simulink model "P2PHVDCMMC"  (R2024a)
settings: Solver=FixedStepDiscrete  StartTime=0.0  StopTime=10  RelTol=1e-3
PreLoadFcn:
  | % HVDCMMCInterconnectionParam
StartFcn:
  | tic
StopFcn:
  | toc
values from neighbouring files (symbols this model uses):
  C_PM = 1.758e-3    (= 0.001758)    [P2PHVDCMMCcode.m]    (also in SFu.mat)
  Cg = 50e-9    (= 5e-08)    [P2PHVDCMMCcode.m]    (also in SFu.mat)
  Fc = Fnom*3.37    (= 168.5)    [P2PHVDCMMCcode.m]    (also in SFu.mat)
  Fnom = 50    [P2PHVDCMMCcode.m]    (also in SFu.mat)
  HRM = 1    [SFu.mat]
  Ki_Ireg = 6    [P2PHVDCMMCcode.m]    (also in SFu.mat)
  Ki_Preg = 1.0    (= 1)    [P2PHVDCMMCcode.m]    (also in SFu.mat)
  Ki_Qreg = 1.0    (= 1)    [P2PHVDCMMCcode.m]    (also in SFu.mat)
  Ki_VDCreg = 100    [P2PHVDCMMCcode.m]    (also in SFu.mat)
  Kp_Ireg = 0.6    [P2PHVDCMMCcode.m]    (also in SFu.mat)
  Kp_Preg = 0.5/3    (= 0.166666666667)    [P2PHVDCMMCcode.m]    (also in SFu.mat)
  Kp_Qreg = 0.5/3    (= 0.166666666667)    [P2PHVDCMMCcode.m]    (also in SFu.mat)
  Kp_VDCreg = 4    [P2PHVDCMMCcode.m]    (also in SFu.mat)
  L_cable = 15e-3    (= 0.015)    [P2PHVDCMMCcode.m]    (also in SFu.mat)
  Larm = Larm_pu*(Zb_ac/(2*pi*Fnom))    [P2PHVDCMMCcode.m]    (also in SFu.mat = 0.0529455974536)
  Larm_pu = 0.15    [P2PHVDCMMCcode.m]    (also in SFu.mat)
  Lff = Larm_pu/2    (= 0.075)    [P2PHVDCMMCcode.m]    (also in SFu.mat)
  Limits_Ireg = [ 2.0  -2.0]    [P2PHVDCMMCcode.m]    (also in SFu.mat = [2 -2])
  Limits_Preg = [ 1.2, 0.8 ]    [P2PHVDCMMCcode.m]    (also in SFu.mat = [1.2 0.8])
  Limits_Qreg = [ 0.25, -0.25 ]    [P2PHVDCMMCcode.m]    (also in SFu.mat = [0.25 -0.25])
  Limits_VDCreg = [ 2.0  -2.0]    [P2PHVDCMMCcode.m]    (also in SFu.mat = [2 -2])
  Lxfo = 0.12    [P2PHVDCMMCcode.m]    (also in SFu.mat)
  N = 1    [P2PHVDCMMCcode.m]    (also in SFu.mat)
  Nb_PM = 36    [P2PHVDCMMCcode.m]    (also in SFu.mat)
  Pnom = 1000e6    (= 1000000000)    [P2PHVDCMMCcode.m]    (also in SFu.mat)
  R_cable = 0.5    [P2PHVDCMMCcode.m]    (also in SFu.mat)
  R_startup = 400    [P2PHVDCMMCcode.m]    (also in SFu.mat)
  Rarm = Rarm_pu*Zb_ac    [P2PHVDCMMCcode.m]    (also in SFu.mat = 0.1663335)
  Rff = Rarm_pu/2    (= 0.00075)    [P2PHVDCMMCcode.m]    (also in SFu.mat)
  Rg = 100    [P2PHVDCMMCcode.m]    (also in SFu.mat)
  Rxfo = 0.003    [P2PHVDCMMCcode.m]    (also in SFu.mat)
  S =     [SFu.mat]
  Slope_Qref = 0.5    [P2PHVDCMMCcode.m]    (also in SFu.mat)
  Slope_Vdc_ref = Vnom_dc/5    (= 128000)    [P2PHVDCMMCcode.m]    (also in SFu.mat)
  Tfault = 9999    [SFu.mat]
  Ts = Ts_Control    (= 4e-05)    [P2PHVDCMMCcode.m]    (also in SFu.mat)
  Ts_Control = 40e-6    (= 4e-05)    [P2PHVDCMMCcode.m]    (also in SFu.mat)
  Ts_dqn = 2e-5    (= 2e-05)    [P2PHVDCMMCcode.m]    (also in SFu.mat)
  Ts_Power = 20e-6    (= 2e-05)    [P2PHVDCMMCcode.m]    (also in SFu.mat)
  Vnom_dc = 640e3    (= 640000)    [P2PHVDCMMCcode.m]    (also in SFu.mat)
  Vnom_prim = 400e3    (= 400000)    [P2PHVDCMMCcode.m]    (also in SFu.mat)
  Vnom_sec = 333e3    (= 333000)    [P2PHVDCMMCcode.m]    (also in SFu.mat)
  Ws = 314.159265359    [SFu.mat]
undefined symbols (not defined in the file or in its folder): DiscIntNeverNeededParam, Discrete, DQN_Lib, gcbh, Int_DQNc_Mat, Mult_DQNc_Mat, Pcc, sps, sps_rtmsupport, spsMeanValueVariableFrequencyModel, spsPLL3phModel, SY3
libraries: simulink x38, spsControlledVoltageSourceLib x30, spsVoltageMeasurementLib x21, spsIdealSwitchLib x21, powerlib_extras x12, spsSecondOrderFilterLib x12, spsCurrentMeasurementLib x12, spsdq0toabcLib x9, spsMeanLib x8, spsMeanVariableFrequencyLib x8, spsabctodq0Lib x8, spsThreePhaseSeriesRLCBranchLib x7
(part 8 of 13)

== system P2PHVDCMMC/Control _DQn_inv/PLL, Measurements and Transformation1/PLL (3ph)2/Model/Variable Frequency Mean value/Model ==
  Freq : Inport  PortDimensions=1
  vq : Inport  Port=2
  Constant : Constant  Value=1/sps.Finit
  Correction subsystem : Subsystem
  Digital Clock : DigitalClock  SampleTime=Ts
  Discrete Variable Time Delay : spsDiscreteVariableTimeDelayLib/Discrete Variable Time Delay  MaxDelay=1/sps.Fmin+Ts  InitialValue=0  Ts=Ts  DFT=on
  Gain : Gain  Gain=Ts  SaturateOnIntegerOverflow=on  OutDataTypeStr=Inherit: Same as input  ParamDataTypeStr=Inherit: Same as input
  Integ4 : DiscreteIntegrator  IntegratorMethod=Integration: Trapezoidal  SampleTime=Ts  ICPrevOutput=DiscIntNeverNeededParam  ICPrevScaledInput=DiscIntNeverNeededParam
  Number of samples per cycle : Fcn  Expr=1/u[1]/Ts
  Product : Product  InputSameDT=on  SaturateOnIntegerOverflow=on  OutDataTypeStr=Inherit: Same as first input
  Relational Operator : RelationalOperator  OutDataTypeStr=boolean  SampleTime=Ts  InputSameDT=off
  Rounding Function : Rounding  Operator=ceil
  Sum5 : Sum  InputSameDT=on  SaturateOnIntegerOverflow=on  OutDataTypeStr=Inherit: Same as first input
  Sum7 : Sum  Inputs=-+  InputSameDT=on  SaturateOnIntegerOverflow=on  OutDataTypeStr=Inherit: Same as first input
  Switch : Switch  Threshold=0.5  SaturateOnIntegerOverflow=off
  To avoid division by zero : Saturate  UpperLimit=1e6  LowerLimit=eps
  Unit Delay1 : UnitDelay  InitialCondition=sps.Vinit  SampleTime=Ts  HasFrameUpgradeWarning=on
  Mean : Outport
  wires:
  Correction subsystem/1(Out) -> Sum5/2
  To avoid division by zero/1 -> Number of samples per cycle/1  "Freq"
  Switch/1 -> Mean/1, Unit Delay1/1
  Sum5/1 -> Switch/1
  Number of samples per cycle/1 -> Correction subsystem/1(N), Rounding Function/1
  Rounding Function/1 -> Correction subsystem/2(F), Gain/1
  Gain/1 -> Discrete Variable Time Delay/2  "Delay"
  Freq/1 -> To avoid division by zero/1, Product/2
  Integ4/1 -> Sum7/2, Discrete Variable Time Delay/1
  Sum7/1 -> Product/1
  Discrete Variable Time Delay/1 -> Sum7/1
  Product/1 -> Sum5/1  "Mean value"
  vq/1 -> Correction subsystem/3(In), Integ4/1
  Digital Clock/1 -> Relational Operator/1
  Unit Delay1/1 -> Switch/3
  Relational Operator/1 -> Switch/2
  Constant/1 -> Relational Operator/2

== system P2PHVDCMMC/Control _DQn_rec/PLL, Measurements and Transformation1/PLL (3ph)/Model/Automatic Gain Control/Positive-Sequence (PLL-Driven) ==
  Freq : Inport  SampleTime=Ts
  dq : Inport  Port=2  SampleTime=Ts
  Complex to Magnitude-Angle : ComplexToMagnitudeAngle
  Mean (Variable Frequency)1 : spsMeanVariableFrequencyLib/Mean (Variable Frequency)  Finit=sps.Finit  Fmin=sps.Fmin  Vinit=sps.Real_Init  Ts=Ts
      settings: LibrarySourceBlock=|
      | sps_lib/Sensors and Measurements/Mean
      | (Variable Frequency)
  Mean (Variable Frequency)2 : spsMeanVariableFrequencyLib/Mean (Variable Frequency)  Finit=sps.Finit  Fmin=sps.Fmin  Vinit=sps.Imag_Init  Ts=Ts
      settings: LibrarySourceBlock=|
      | sps_lib/Sensors and Measurements/Mean
      | (Variable Frequency)
  Rad->Deg. : Gain  Gain=180/pi  SaturateOnIntegerOverflow=on  OutDataTypeStr=Inherit: Same as input  ParamDataTypeStr=Inherit: Same as input
  Real-Imag to Complex : RealImagToComplex
  Selector : Selector  InputPortWidth=2  IndexOptions=Index vector (dialog)  Indices=[1]  OutputSizes=1
  Selector1 : Selector  InputPortWidth=2  IndexOptions=Index vector (dialog)  Indices=[2]  OutputSizes=1
  Mag : Outport  SampleTime=Ts  VectorParamsAs1DForOutWhenUnconnected=off
  Phase : Outport  Port=2  SampleTime=Ts  VectorParamsAs1DForOutWhenUnconnected=off
  wires:
  Rad->Deg./1 -> Phase/1
  Mean (Variable Frequency)1/1 -> Real-Imag to Complex/1
  Freq/1 -> Mean (Variable Frequency)1/1, Mean (Variable Frequency)2/1
  Real-Imag to Complex/1 -> Complex to Magnitude-Angle/1
  Mean (Variable Frequency)2/1 -> Real-Imag to Complex/2
  Complex to Magnitude-Angle/1 -> Mag/1
  Complex to Magnitude-Angle/2 -> Rad->Deg./1
  dq/1 -> Selector/1, Selector1/1  "q"
  Selector/1 -> Mean (Variable Frequency)1/2  "d"
  Selector1/1 -> Mean (Variable Frequency)2/2  "q"

== system P2PHVDCMMC/Control _DQn_rec/PLL, Measurements and Transformation1/PLL (3ph)/Model/Variable Frequency Mean value/Model ==
  Freq : Inport  PortDimensions=1
  vq : Inport  Port=2
  Constant : Constant  Value=1/sps.Finit
  Correction subsystem : Subsystem
  Digital Clock : DigitalClock  SampleTime=Ts
  Discrete Variable Time Delay : spsDiscreteVariableTimeDelayLib/Discrete Variable Time Delay  MaxDelay=1/sps.Fmin+Ts  InitialValue=0  Ts=Ts  DFT=on
  Gain : Gain  Gain=Ts  SaturateOnIntegerOverflow=on  OutDataTypeStr=Inherit: Same as input  ParamDataTypeStr=Inherit: Same as input
  Integ4 : DiscreteIntegrator  IntegratorMethod=Integration: Trapezoidal  SampleTime=Ts  ICPrevOutput=DiscIntNeverNeededParam  ICPrevScaledInput=DiscIntNeverNeededParam
  Number of samples per cycle : Fcn  Expr=1/u[1]/Ts
  Product : Product  InputSameDT=on  SaturateOnIntegerOverflow=on  OutDataTypeStr=Inherit: Same as first input
  Relational Operator : RelationalOperator  OutDataTypeStr=boolean  SampleTime=Ts  InputSameDT=off
  Rounding Function : Rounding  Operator=ceil
  Sum5 : Sum  InputSameDT=on  SaturateOnIntegerOverflow=on  OutDataTypeStr=Inherit: Same as first input
  Sum7 : Sum  Inputs=-+  InputSameDT=on  SaturateOnIntegerOverflow=on  OutDataTypeStr=Inherit: Same as first input
  Switch : Switch  Threshold=0.5  SaturateOnIntegerOverflow=off
  To avoid division by zero : Saturate  UpperLimit=1e6  LowerLimit=eps
  Unit Delay1 : UnitDelay  InitialCondition=sps.Vinit  SampleTime=Ts  HasFrameUpgradeWarning=on
  Mean : Outport
  wires:
  Correction subsystem/1(Out) -> Sum5/2
  To avoid division by zero/1 -> Number of samples per cycle/1  "Freq"
  Switch/1 -> Mean/1, Unit Delay1/1
  Sum5/1 -> Switch/1
  Number of samples per cycle/1 -> Correction subsystem/1(N), Rounding Function/1
  Rounding Function/1 -> Correction subsystem/2(F), Gain/1
  Gain/1 -> Discrete Variable Time Delay/2  "Delay"
  Freq/1 -> To avoid division by zero/1, Product/2
  Integ4/1 -> Sum7/2, Discrete Variable Time Delay/1
  Sum7/1 -> Product/1
  Discrete Variable Time Delay/1 -> Sum7/1
  Product/1 -> Sum5/1  "Mean value"
  vq/1 -> Correction subsystem/3(In), Integ4/1
  Digital Clock/1 -> Relational Operator/1
  Unit Delay1/1 -> Switch/3
  Relational Operator/1 -> Switch/2
  Constant/1 -> Relational Operator/2

== system P2PHVDCMMC/Control _DQn_rec/PLL, Measurements and Transformation1/PLL (3ph)2/Model/Automatic Gain Control/Positive-Sequence (PLL-Driven) ==
  Freq : Inport  SampleTime=Ts
  dq : Inport  Port=2  SampleTime=Ts
  Complex to Magnitude-Angle : ComplexToMagnitudeAngle
  Mean (Variable Frequency)1 : spsMeanVariableFrequencyLib/Mean (Variable Frequency)  Finit=sps.Finit  Fmin=sps.Fmin  Vinit=sps.Real_Init  Ts=Ts
      settings: LibrarySourceBlock=|
      | sps_lib/Sensors and Measurements/Mean
      | (Variable Frequency)
  Mean (Variable Frequency)2 : spsMeanVariableFrequencyLib/Mean (Variable Frequency)  Finit=sps.Finit  Fmin=sps.Fmin  Vinit=sps.Imag_Init  Ts=Ts
      settings: LibrarySourceBlock=|
      | sps_lib/Sensors and Measurements/Mean
      | (Variable Frequency)
  Rad->Deg. : Gain  Gain=180/pi  SaturateOnIntegerOverflow=on  OutDataTypeStr=Inherit: Same as input  ParamDataTypeStr=Inherit: Same as input
  Real-Imag to Complex : RealImagToComplex
  Selector : Selector  InputPortWidth=2  IndexOptions=Index vector (dialog)  Indices=[1]  OutputSizes=1
  Selector1 : Selector  InputPortWidth=2  IndexOptions=Index vector (dialog)  Indices=[2]  OutputSizes=1
  Mag : Outport  SampleTime=Ts  VectorParamsAs1DForOutWhenUnconnected=off
  Phase : Outport  Port=2  SampleTime=Ts  VectorParamsAs1DForOutWhenUnconnected=off
  wires:
  Rad->Deg./1 -> Phase/1
  Mean (Variable Frequency)1/1 -> Real-Imag to Complex/1
  Freq/1 -> Mean (Variable Frequency)1/1, Mean (Variable Frequency)2/1
  Real-Imag to Complex/1 -> Complex to Magnitude-Angle/1
  Mean (Variable Frequency)2/1 -> Real-Imag to Complex/2
  Complex to Magnitude-Angle/1 -> Mag/1
  Complex to Magnitude-Angle/2 -> Rad->Deg./1
  dq/1 -> Selector/1, Selector1/1  "q"
  Selector/1 -> Mean (Variable Frequency)1/2  "d"
  Selector1/1 -> Mean (Variable Frequency)2/2  "q"

== system P2PHVDCMMC/Control _DQn_rec/PLL, Measurements and Transformation1/PLL (3ph)2/Model/Variable Frequency Mean value/Model ==
  Freq : Inport  PortDimensions=1
  vq : Inport  Port=2
  Constant : Constant  Value=1/sps.Finit
  Correction subsystem : Subsystem
  Digital Clock : DigitalClock  SampleTime=Ts
  Discrete Variable Time Delay : spsDiscreteVariableTimeDelayLib/Discrete Variable Time Delay  MaxDelay=1/sps.Fmin+Ts  InitialValue=0  Ts=Ts  DFT=on
  Gain : Gain  Gain=Ts  SaturateOnIntegerOverflow=on  OutDataTypeStr=Inherit: Same as input  ParamDataTypeStr=Inherit: Same as input
  Integ4 : DiscreteIntegrator  IntegratorMethod=Integration: Trapezoidal  SampleTime=Ts  ICPrevOutput=DiscIntNeverNeededParam  ICPrevScaledInput=DiscIntNeverNeededParam
  Number of samples per cycle : Fcn  Expr=1/u[1]/Ts
  Product : Product  InputSameDT=on  SaturateOnIntegerOverflow=on  OutDataTypeStr=Inherit: Same as first input
  Relational Operator : RelationalOperator  OutDataTypeStr=boolean  SampleTime=Ts  InputSameDT=off
  Rounding Function : Rounding  Operator=ceil
  Sum5 : Sum  InputSameDT=on  SaturateOnIntegerOverflow=on  OutDataTypeStr=Inherit: Same as first input
  Sum7 : Sum  Inputs=-+  InputSameDT=on  SaturateOnIntegerOverflow=on  OutDataTypeStr=Inherit: Same as first input
  Switch : Switch  Threshold=0.5  SaturateOnIntegerOverflow=off
  To avoid division by zero : Saturate  UpperLimit=1e6  LowerLimit=eps
  Unit Delay1 : UnitDelay  InitialCondition=sps.Vinit  SampleTime=Ts  HasFrameUpgradeWarning=on
  Mean : Outport
  wires:
  Correction subsystem/1(Out) -> Sum5/2
  To avoid division by zero/1 -> Number of samples per cycle/1  "Freq"
  Switch/1 -> Mean/1, Unit Delay1/1
  Sum5/1 -> Switch/1
  Number of samples per cycle/1 -> Correction subsystem/1(N), Rounding Function/1
  Rounding Function/1 -> Correction subsystem/2(F), Gain/1
  Gain/1 -> Discrete Variable Time Delay/2  "Delay"
  Freq/1 -> To avoid division by zero/1, Product/2
  Integ4/1 -> Sum7/2, Discrete Variable Time Delay/1
  Sum7/1 -> Product/1
  Discrete Variable Time Delay/1 -> Sum7/1
  Product/1 -> Sum5/1  "Mean value"
  vq/1 -> Correction subsystem/3(In), Integ4/1
  Digital Clock/1 -> Relational Operator/1
  Unit Delay1/1 -> Switch/3
  Relational Operator/1 -> Switch/2
  Constant/1 -> Relational Operator/2

== system P2PHVDCMMC/Control _DQn_inv/PLL, Measurements and Transformation1/PLL (3ph)/Model/Variable Frequency Mean value/Model/Correction subsystem ==
  N : Inport
  F : Inport  Port=2
  In : Inport  Port=3
  Gain1 : Gain  Gain=0.5  SaturateOnIntegerOverflow=on  OutDataTypeStr=Inherit: Same as input  ParamDataTypeStr=Inherit: Same as input
  Product2 : Product  Inputs=*/  InputSameDT=on  SaturateOnIntegerOverflow=on  OutDataTypeStr=Inherit: Same as first input
  Product4 : Product  Inputs=**  InputSameDT=on  SaturateOnIntegerOverflow=on  OutDataTypeStr=Inherit: Same as first input
  Product5 : Product  Inputs=**  InputSameDT=on  SaturateOnIntegerOverflow=on  OutDataTypeStr=Inherit: Same as first input
  Sum1 : Sum  Inputs=+-  InputSameDT=on  SaturateOnIntegerOverflow=on  OutDataTypeStr=Inherit: Same as first input
  Sum4 : Sum  InputSameDT=on  SaturateOnIntegerOverflow=on  OutDataTypeStr=Inherit: Same as first input
  Sum5 : Sum  Inputs=+-  InputSameDT=on  SaturateOnIntegerOverflow=on  OutDataTypeStr=Inherit: Same as first input
  Unit Delay : UnitDelay  SampleTime=Ts  HasFrameUpgradeWarning=on
  Out : Outport
  wires:
  Product4/1 -> Out/1
  Sum4/1 -> Product4/2
  Gain1/1 -> Sum4/1
  Product5/1 -> Gain1/1
  Sum1/1 -> Product5/2
  In/1 -> Sum4/2, Unit Delay/1, Sum1/1
  Product2/1 -> Product4/1
  Sum5/1 -> Product5/1, Product2/1
  F/1 -> Sum5/2
  N/1 -> Product2/2, Sum5/1
  Unit Delay/1 -> Sum1/2

== system P2PHVDCMMC/Control _DQn_inv/PLL, Measurements and Transformation1/PLL (3ph)2/Model/Variable Frequency Mean value/Model/Correction subsystem ==
  N : Inport
  F : Inport  Port=2
  In : Inport  Port=3
  Gain1 : Gain  Gain=0.5  SaturateOnIntegerOverflow=on  OutDataTypeStr=Inherit: Same as input  ParamDataTypeStr=Inherit: Same as input
  Product2 : Product  Inputs=*/  InputSameDT=on  SaturateOnIntegerOverflow=on  OutDataTypeStr=Inherit: Same as first input
  Product4 : Product  Inputs=**  InputSameDT=on  SaturateOnIntegerOverflow=on  OutDataTypeStr=Inherit: Same as first input
  Product5 : Product  Inputs=**  InputSameDT=on  SaturateOnIntegerOverflow=on  OutDataTypeStr=Inherit: Same as first input
  Sum1 : Sum  Inputs=+-  InputSameDT=on  SaturateOnIntegerOverflow=on  OutDataTypeStr=Inherit: Same as first input
  Sum4 : Sum  InputSameDT=on  SaturateOnIntegerOverflow=on  OutDataTypeStr=Inherit: Same as first input
  Sum5 : Sum  Inputs=+-  InputSameDT=on  SaturateOnIntegerOverflow=on  OutDataTypeStr=Inherit: Same as first input
  Unit Delay : UnitDelay  SampleTime=Ts  HasFrameUpgradeWarning=on
  Out : Outport
  wires:
  Product4/1 -> Out/1
  Sum4/1 -> Product4/2
  Gain1/1 -> Sum4/1
  Product5/1 -> Gain1/1
  Sum1/1 -> Product5/2
  In/1 -> Sum4/2, Unit Delay/1, Sum1/1
  Product2/1 -> Product4/1
  Sum5/1 -> Product5/1, Product2/1
  F/1 -> Sum5/2
  N/1 -> Product2/2, Sum5/1
  Unit Delay/1 -> Sum1/2

== system P2PHVDCMMC/Control _DQn_rec/PLL, Measurements and Transformation1/PLL (3ph)/Model/Variable Frequency Mean value/Model/Correction subsystem ==
  N : Inport
  F : Inport  Port=2
  In : Inport  Port=3
  Gain1 : Gain  Gain=0.5  SaturateOnIntegerOverflow=on  OutDataTypeStr=Inherit: Same as input  ParamDataTypeStr=Inherit: Same as input
  Product2 : Product  Inputs=*/  InputSameDT=on  SaturateOnIntegerOverflow=on  OutDataTypeStr=Inherit: Same as first input
  Product4 : Product  Inputs=**  InputSameDT=on  SaturateOnIntegerOverflow=on  OutDataTypeStr=Inherit: Same as first input
  Product5 : Product  Inputs=**  InputSameDT=on  SaturateOnIntegerOverflow=on  OutDataTypeStr=Inherit: Same as first input
  Sum1 : Sum  Inputs=+-  InputSameDT=on  SaturateOnIntegerOverflow=on  OutDataTypeStr=Inherit: Same as first input
  Sum4 : Sum  InputSameDT=on  SaturateOnIntegerOverflow=on  OutDataTypeStr=Inherit: Same as first input
  Sum5 : Sum  Inputs=+-  InputSameDT=on  SaturateOnIntegerOverflow=on  OutDataTypeStr=Inherit: Same as first input
  Unit Delay : UnitDelay  SampleTime=Ts  HasFrameUpgradeWarning=on
  Out : Outport
  wires:
  Product4/1 -> Out/1
  Sum4/1 -> Product4/2
  Gain1/1 -> Sum4/1
  Product5/1 -> Gain1/1
  Sum1/1 -> Product5/2
  In/1 -> Sum4/2, Unit Delay/1, Sum1/1
  Product2/1 -> Product4/1
  Sum5/1 -> Product5/1, Product2/1
  F/1 -> Sum5/2
  N/1 -> Product2/2, Sum5/1
  Unit Delay/1 -> Sum1/2

== system P2PHVDCMMC/Control _DQn_rec/PLL, Measurements and Transformation1/PLL (3ph)2/Model/Variable Frequency Mean value/Model/Correction subsystem ==
  N : Inport
  F : Inport  Port=2
  In : Inport  Port=3
  Gain1 : Gain  Gain=0.5  SaturateOnIntegerOverflow=on  OutDataTypeStr=Inherit: Same as input  ParamDataTypeStr=Inherit: Same as input
  Product2 : Product  Inputs=*/  InputSameDT=on  SaturateOnIntegerOverflow=on  OutDataTypeStr=Inherit: Same as first input
  Product4 : Product  Inputs=**  InputSameDT=on  SaturateOnIntegerOverflow=on  OutDataTypeStr=Inherit: Same as first input
  Product5 : Product  Inputs=**  InputSameDT=on  SaturateOnIntegerOverflow=on  OutDataTypeStr=Inherit: Same as first input
  Sum1 : Sum  Inputs=+-  InputSameDT=on  SaturateOnIntegerOverflow=on  OutDataTypeStr=Inherit: Same as first input
  Sum4 : Sum  InputSameDT=on  SaturateOnIntegerOverflow=on  OutDataTypeStr=Inherit: Same as first input
  Sum5 : Sum  Inputs=+-  InputSameDT=on  SaturateOnIntegerOverflow=on  OutDataTypeStr=Inherit: Same as first input
  Unit Delay : UnitDelay  SampleTime=Ts  HasFrameUpgradeWarning=on
  Out : Outport
  wires:
  Product4/1 -> Out/1
  Sum4/1 -> Product4/2
  Gain1/1 -> Sum4/1
  Product5/1 -> Gain1/1
  Sum1/1 -> Product5/2
  In/1 -> Sum4/2, Unit Delay/1, Sum1/1
  Product2/1 -> Product4/1
  Sum5/1 -> Product5/1, Product2/1
  F/1 -> Sum5/2
  N/1 -> Product2/2, Sum5/1
  Unit Delay/1 -> Sum1/2

== matlab function P2PHVDCMMC/Subsystem4/ACrec/Mult_DQNc_Mat2 ==
  data: Xdcpnz_c input; Ydcpnz_c input; N parameter; HrmDbl parameter; Zdcpnz_c output
function Zdcpnz_c    = fMultDQNc(Xdcpnz_c, Ydcpnz_c, N, HrmDbl)
    Zdcpnz_c = complex(zeros(3,2*N+1));

    persistent T132;
    persistent T213;
    persistent T231;
    persistent T321;
    persistent T312;
    persistent Sas;
    persistent Ssa;

    if(isempty(T132)) 
        T132 = [1 0 0; 0 0 1; 0 1 0];
        T213 = [0 1 0; 1 0 0; 0 0 1];
        T231 = [0 1 0; 0 0 1; 1 0 0];
        T321 = [0 0 1; 0 1 0; 1 0 0];
        T312 = [0 0 1; 1 0 0; 0 1 0];

        a = -0.5+0.866i;
        a2 = -0.5-0.866i;
        Sas = [1,a,a2;1,a2,a;1,1,1]/3;
        Ssa = eye(3)/(Sas);
    end

%%%%%%%%%%%%%%%%%%%%%%%%%%%%%%

    Zdcpnz_c(:,1) = Sas*(Ssa*Xdcpnz_c(:,1).*Ssa*Ydcpnz_c(:,1));

    sX = size(Xdcpnz_c,2);
    Xdcpnz_c = [Xdcpnz_c zeros(3,N+1-sX)];

    sY = size(Ydcpnz_c,2);
    Ydcpnz_c = [Ydcpnz_c zeros(3,N+1-sY)];

       
    for h = 1 : 2*N
        if(h<=N)

            Zdcpnz_c(3,1) = Zdcpnz_c(3,1) + 0.5*real(Xdcpnz_c(:,h+1)'*Ydcpnz_c(:,h+1));


            Zdcpnz_c(3,2*h+1) = Zdcpnz_c(3,2*h+1) + 0.5*Xdcpnz_c(1,h+1)*Ydcpnz_c(2,h+1)*exp(-1i*pi/2);

            Zdcpnz_c(1:2,1) = Zdcpnz_c(1:2,1) + 0.25*abs(Xdcpnz_c(1,h+1))*abs(Ydcpnz_c(2,h+1))*[1;1].*exp(1i*((-angle(Xdcpnz_c(1,h+1))+angle(Ydcpnz_c(2,h+1)))*[1;-1]));
            Zdcpnz_c(1:2,1) = Zdcpnz_c(1:2,1) + 0.25*abs(Xdcpnz_c(1,h+1))*abs(Ydcpnz_c(3,h+1))*[1;1].*exp(1i*((-angle(Xdcpnz_c(1,h+1))+angle(Ydcpnz_c(3,h+1)))*[-1;1]));


            Zdcpnz_c(3,2*h+1) = Zdcpnz_c(3,2*h+1) + 0.5*Xdcpnz_c(2,h+1)*Ydcpnz_c(1,h+1)*exp(-1i*pi/2);


            Zdcpnz_c(1:2,1) = Zdcpnz_c(1:2,1) + 0.25*abs(Xdcpnz_c(2,h+1))*abs(Ydcpnz_c(1,h+1))*[1;1].*exp(1i*((-angle(Xdcpnz_c(2,h+1))+angle(Ydcpnz_c(1,h+1)))*[-1;1]));
            Zdcpnz_c(1:2,1) = Zdcpnz_c(1:2,1) + 0.25*abs(Xdcpnz_c(2,h+1))*abs(Ydcpnz_c(3,h+1))*[1;1].*exp(1i*((-angle(Xdcpnz_c(2,h+1))+angle(Ydcpnz_c(3,h+1)))*[1;-1]));
            
            Zdcpnz_c(1:2,1) = Zdcpnz_c(1:2,1) + 0.25*abs(Xdcpnz_c(3,h+1))*abs(Ydcpnz_c(1,h+1))*[1;1].*exp(1i*((-angle(Xdcpnz_c(3,h+1))+angle(Ydcpnz_c(1,h+1)))*[1;-1]));
            Zdcpnz_c(1:2,1) = Zdcpnz_c(1:2,1) + 0.25*abs(Xdcpnz_c(3,h+1))*abs(Ydcpnz_c(2,h+1))*[1;1].*exp(1i*((-angle(Xdcpnz_c(3,h+1))+angle(Ydcpnz_c(2,h+1)))*[-1;+1]));

            %%%%%%%%%%%%%%%%% POSITIVE (Ydc*Xp) %%%%%%%%%%%%%%%%%%%
            Zdcpnz_c(:,h+1) = Zdcpnz_c(:,h+1) + T312*Ydcpnz_c(:,1)*Xdcpnz_c(1,h+1); %[0 0 1; 1 0 0; 0 1 0]
            %%%%%%%%%%%%%%%%% POSITIVE (Xdc*Yp) %%%%%%%%%%%%%%%%%%%
            Zdcpnz_c(:,h+1) = Zdcpnz_c(:,h+1) + T312*Xdcpnz_c(:,1)*Ydcpnz_c(1,h+1);
            %%%%%%%%%%%%%%%%% NEGATIVE (Ydc*Xn) %%%%%%%%%%%%%%%%%%%
            Zdcpnz_c(:,h+1) = Zdcpnz_c(:,h+1) + T231*Ydcpnz_c(:,1)*Xdcpnz_c(2,h+1);
            %%%%%%%%%%%%%%%%% NEGATIVE (Xdc*Yn) %%%%%%%%%%%%%%%%%%%
            Zdcpnz_c(:,h+1) = Zdcpnz_c(:,h+1) + T231*Xdcpnz_c(:,1)*Ydcpnz_c(2,h+1);
            %%%%%%%%%%%%%%%%%%%%%%%%%%%%%%%%%%%%%%%%%%%%%%%%%%%%%%
            Zdcpnz_c(:,h+1) = Zdcpnz_c(:,h+1) + Ydcpnz_c(:,1)*Xdcpnz_c(3,h+1);
            %%%%%%%%%%%%%%%%%%%%%%%%%%%%%%%%%%%%%%%%%%%%%%%%%%%%%%
            Zdcpnz_c(:,h+1) = Zdcpnz_c(:,h+1) + Xdcpnz_c(:,1)*Ydcpnz_c(3,h+1);
            
%%%%%%%%%%%%%%%%%%%%%% h<=N ODD %%%%%%%%%%%%%%%%%%%%%%%%%%%%%%%%%%%%%%%%%
            if(mod(h,2)==1) 
                %%%%%%%%%%%%%%%%% D3p (3ph+) %%%%%%%%%%%%%%%%%%%%%%%

                %&%%%%%%%%%%%%%%%%%%%%%%%%%% PP + NN %%%%%%%%%%%%%%%%%%%%%%%%%%%
                for i = 1 : h - 1
                   Zdcpnz_c(1,h+1) = Zdcpnz_c(1,h+1) +    0.5*( real(Xdcpnz_c(2,i+1))*imag(Ydcpnz_c(2,h-i+1)) + imag(Xdcpnz_c(2,i+1))*real(Ydcpnz_c(2,h-i+1)) );
                   Zdcpnz_c(1,h+1) = Zdcpnz_c(1,h+1) + 1i*0.5*( -real(Xdcpnz_c(2,i+1))*real(Ydcpnz_c(2,h-i+1)) + imag(Xdcpnz_c(2,i+1))*imag(Ydcpnz_c(2,h-i+1)) );

                   Zdcpnz_c(2,h+1) = Zdcpnz_c(2,h+1) +    0.5*( real(Xdcpnz_c(1,i+1))*imag(Ydcpnz_c(1,h-i+1)) + imag(Xdcpnz_c(1,i+1))*real(Ydcpnz_c(1,h-i+1)) );
                   Zdcpnz_c(2,h+1) = Zdcpnz_c(2,h+1) + 1i*0.5*( -real(Xdcpnz_c(1,i+1))*real(Ydcpnz_c(1,h-i+1)) + imag(Xdcpnz_c(1,i+1))*imag(Ydcpnz_c(1,h-i+1)) );
                end

                for i = 1 : N - h

                    Zdcpnz_c(3,h+1) = Zdcpnz_c(3,h+1) -    imag(0.5*Xdcpnz_c(1:2,i+1)'*Ydcpnz_c(1:2,i+h+1)) -    imag(0.5*Ydcpnz_c(1:2,i+1)'*Xdcpnz_c(1:2,i+h+1));
                    Zdcpnz_c(3,h+1) = Zdcpnz_c(3,h+1) + 1i*real(0.5*Xdcpnz_c(1:2,i+1)'*Ydcpnz_c(1:2,i+h+1)) + 1i*real(0.5*Ydcpnz_c(1:2,i+1)'*Xdcpnz_c(1:2,i+h+1));

                end
                %&%%%%%%%%%%%%%%%%%%%%%%%%%% PP + NN %%%%%%%%%%%%%%%%%%%%%%%%%%%

                for k = 1 : (N + mod(N+1,2) - h)/2
                    i = 2*k-1;
                    j = i+h;

                    Zdcpnz_c(1,h+1) = Zdcpnz_c(1,h+1) + (0.5*(Xdcpnz_c(:,i+1)'*T132*T213*Ydcpnz_c(:,j+1))*exp(+1i*pi/2)) ...
                                                      + (0.5*(Xdcpnz_c(:,j+1)'*T213*T132*Ydcpnz_c(:,i+1))*exp(-1i*pi/2))';

                    Zdcpnz_c(2,h+1) = Zdcpnz_c(2,h+1) + (0.5*(Xdcpnz_c(:,i+1)'*T132*T321*Ydcpnz_c(:,j+1))*exp(+1i*pi/2)) ...
                                                      + (0.5*(Xdcpnz_c(:,j+1)'*T321*T132*Ydcpnz_c(:,i+1))*exp(-1i*pi/2))';

                    Zdcpnz_c(3,h+1) = Zdcpnz_c(3,h+1) + (0.5*Xdcpnz_c(3,i+1)'*Ydcpnz_c(3,j+1)*exp(1i*pi/2)) ...
                                                      - (0.5*Xdcpnz_c(3,j+1)'*Ydcpnz_c(3,i+1)*exp(1i*pi/2))';
                end

                for k = 1 : (N + mod(N,2) - h - 1)/2
                    i = 2*k;
                    j = i+h;
                    
                    Zdcpnz_c(1,h+1) = Zdcpnz_c(1,h+1) + (0.5*(Xdcpnz_c(:,i+1)'*T132*T213*Ydcpnz_c(:,j+1))*exp(+1i*pi/2)) ...
                                                      + (0.5*(Xdcpnz_c(:,j+1)'*T213*T132*Ydcpnz_c(:,i+1))*exp(-1i*pi/2))';

                    Zdcpnz_c(2,h+1) = Zdcpnz_c(2,h+1) + (0.5*(Xdcpnz_c(:,i+1)'*T132*T321*Ydcpnz_c(:,j+1))*exp(+1i*pi/2)) ...
                                                      + (0.5*(Xdcpnz_c(:,j+1)'*T321*T132*Ydcpnz_c(:,i+1))*exp(-1i*pi/2))';

                    Zdcpnz_c(3,h+1) = Zdcpnz_c(3,h+1) + (0.5*Xdcpnz_c(3,i+1)'*Ydcpnz_c(3,j+1)*exp(1i*pi/2)) ...
                                                      - (0.5*Xdcpnz_c(3,j+1)'*Ydcpnz_c(3,i+1)*exp(1i*pi/2))';
                end

                for k = (h-1)/2:-1:1
                    i = k;
                    j = h-i;  

                    Zdcpnz_c(3,h+1) = Zdcpnz_c(3,h+1) + 0.5*(real(Xdcpnz_c(:,i+1))'*T213*imag(Ydcpnz_c(:,j+1)) + imag(Xdcpnz_c(:,i+1))'*T213*real(Ydcpnz_c(:,j+1)) ...
                                                           + real(Xdcpnz_c(:,j+1))'*T213*imag(Ydcpnz_c(:,i+1)) + imag(Xdcpnz_c(:,j+1))'*T213*real(Ydcpnz_c(:,i+1)));
                                                                                       
                    Zdcpnz_c(3,h+1) = Zdcpnz_c(3,h+1) + 1i*0.5*(-real(Xdcpnz_c(:,i+1))'*T213*real(Ydcpnz_c(:,j+1)) + imag(Xdcpnz_c(:,i+1))'*T213*imag(Ydcpnz_c(:,j+1)) ...
                                                           - real(Xdcpnz_c(:,j+1))'*T213*real(Ydcpnz_c(:,i+1)) + imag(Xdcpnz_c(:,j+1))'*T213*imag(Ydcpnz_c(:,i+1)));

                    Zdcpnz_c(1,h+1) = Zdcpnz_c(1,h+1) + 0.5*(real(Xdcpnz_c([1,3],i+1))'*[0 1; 1 0]*imag(Ydcpnz_c([1,3],j+1)) + imag(Xdcpnz_c([1,3],i+1))'*[0 1; 1 0]*real(Ydcpnz_c([1,3],j+1)) ...
                                                           + real(Xdcpnz_c([1,3],j+1))'*[0 1; 1 0]*imag(Ydcpnz_c([1,3],i+1)) + imag(Xdcpnz_c([1,3],j+1))'*[0 1; 1 0]*real(Ydcpnz_c([1,3],i+1)) );

                    Zdcpnz_c(1,h+1) = Zdcpnz_c(1,h+1) + 1i*0.5*(-real(Xdcpnz_c([1,3],i+1))'*[0 1; 1 0]*real(Ydcpnz_c([1,3],j+1)) + imag(Xdcpnz_c([1,3],i+1))'*[0 1; 1 0]*imag(Ydcpnz_c([1,3],j+1)) ...
                                                              - real(Xdcpnz_c([1,3],j+1))'*[0 1; 1 0]*real(Ydcpnz_c([1,3],i+1)) + imag(Xdcpnz_c([1,3],j+1))'*[0 1; 1 0]*imag(Ydcpnz_c([1,3],i+1)) );

                    Zdcpnz_c(2,h+1) = Zdcpnz_c(2,h+1) + 0.5*(real(Xdcpnz_c([2,3],i+1))'*[0 1; 1 0]*imag(Ydcpnz_c([2,3],j+1)) + imag(Xdcpnz_c([2,3],i+1))'*[0 1; 1 0]*real(Ydcpnz_c([2,3],j+1)) ...
                                                           + real(Xdcpnz_c([2,3],j+1))'*[0 1; 1 0]*imag(Ydcpnz_c([2,3],i+1)) + imag(Xdcpnz_c([2,3],j+1))'*[0 1; 1 0]*real(Ydcpnz_c([2,3],i+1)) );

                    Zdcpnz_c(2,h+1) = Zdcpnz_c(2,h+1) + 1i*0.5*(-real(Xdcpnz_c([2,3],i+1))'*[0 1; 1 0]*real(Ydcpnz_c([2,3],j+1)) + imag(Xdcpnz_c([2,3],i+1))'*[0 1; 1 0]*imag(Ydcpnz_c([2,3],j+1)) ...
                                                              - real(Xdcpnz_c([2,3],j+1))'*[0 1; 1 0]*real(Ydcpnz_c([2,3],i+1)) + imag(Xdcpnz_c([2,3],j+1))'*[0 1; 1 0]*imag(Ydcpnz_c([2,3],i+1)) );

                end
%%%%%%%%%%%%%%%%%%%%%% h<=N EVEN %%%%%%%%%%%%%%%%%%%%%%%%%%%%%%%%%%%%%%%%%           
            else  

                Zdcpnz_c(3,h+1) = Zdcpnz_c(3,h+1) + 0.5*imag(Xdcpnz_c(3,h/2+1)*Ydcpnz_c(3,h/2+1))           -0.5*1i*real(Xdcpnz_c(3,h/2+1)*Ydcpnz_c(3,h/2+1));
                Zdcpnz_c(1,h+1) = Zdcpnz_c(1,h+1) + 0.5*real(Xdcpnz_c(:,h/2+1))'*T321*imag(Ydcpnz_c(:,h/2+1)) + 0.5*imag(Xdcpnz_c(:,h/2+1))'*T321*real(Ydcpnz_c(:,h/2+1));
                Zdcpnz_c(1,h+1) = Zdcpnz_c(1,h+1) - 0.5*1i*real(Xdcpnz_c(:,h/2+1))'*T321*real(Ydcpnz_c(:,h/2+1)) + 0.5*1i*imag(Xdcpnz_c(:,h/2+1))'*T321*imag(Ydcpnz_c(:,h/2+1));
                Zdcpnz_c(2,h+1) = Zdcpnz_c(2,h+1) + 0.5*real(Xdcpnz_c(:,h/2+1))'*T132*imag(Ydcpnz_c(:,h/2+1)) + 0.5*imag(Xdcpnz_c(:,h/2+1))'*T132*real(Ydcpnz_c(:,h/2+1));
                Zdcpnz_c(2,h+1) = Zdcpnz_c(2,h+1) - 0.5*1i*real(Xdcpnz_c(:,h/2+1))'*T132*real(Ydcpnz_c(:,h/2+1)) + 0.5*1i*imag(Xdcpnz_c(:,h/2+1))'*T132*imag(Ydcpnz_c(:,h/2+1));
                
                for k = 1:N-h
                    i = k;
                    j = h+i;

                    Zdcpnz_c(1,h+1) = Zdcpnz_c(1,h+1) + 0.5*( - real(Xdcpnz_c(:,i+1))'*T231*imag(Ydcpnz_c(:,j+1)) + imag(Xdcpnz_c(:,i+1))'*T231*real(Ydcpnz_c(:,j+1)) ...
                                                              + real(Xdcpnz_c(:,j+1))'*T312*imag(Ydcpnz_c(:,i+1)) - imag(Xdcpnz_c(:,j+1))'*T312*real(Ydcpnz_c(:,i+1)));

                    Zdcpnz_c(1,h+1) = Zdcpnz_c(1,h+1) + 0.5*1i*( + real(Xdcpnz_c(:,i+1))'*T231*real(Ydcpnz_c(:,j+1)) + imag(Xdcpnz_c(:,i+1))'*T231*imag(Ydcpnz_c(:,j+1)) ...
                                                                 + real(Xdcpnz_c(:,j+1))'*T312*real(Ydcpnz_c(:,i+1)) + imag(Xdcpnz_c(:,j+1))'*T312*imag(Ydcpnz_c(:,i+1)));

                    Zdcpnz_c(2,h+1) = Zdcpnz_c(2,h+1) + 0.5*( - real(Xdcpnz_c(:,i+1))'*T312*imag(Ydcpnz_c(:,j+1)) + imag(Xdcpnz_c(:,i+1))'*T312*real(Ydcpnz_c(:,j+1)) ...
                                                              + real(Xdcpnz_c(:,j+1))'*T231*imag(Ydcpnz_c(:,i+1)) - imag(Xdcpnz_c(:,j+1))'*T231*real(Ydcpnz_c(:,i+1)));

                    Zdcpnz_c(2,h+1) = Zdcpnz_c(2,h+1) + 1i*0.5*( + real(Xdcpnz_c(:,i+1))'*T312*real(Ydcpnz_c(:,j+1)) + imag(Xdcpnz_c(:,i+1))'*T312*imag(Ydcpnz_c(:,j+1)) ...
                                                              + real(Xdcpnz_c(:,j+1))'*T231*real(Ydcpnz_c(:,i+1)) + imag(Xdcpnz_c(:,j+1))'*T231*imag(Ydcpnz_c(:,i+1)));

                    Zdcpnz_c(3,h+1) = Zdcpnz_c(3,h+1) + 0.5*(-real(Xdcpnz_c(:,i+1))'*imag(Ydcpnz_c(:,j+1))+imag(Xdcpnz_c(:,i+1))'*real(Ydcpnz_c(:,j+1)) ...
                                                             +real(Xdcpnz_c(:,j+1))'*imag(Ydcpnz_c(:,i+1))-imag(Xdcpnz_c(:,j+1))'*real(Ydcpnz_c(:,i+1)));

                    Zdcpnz_c(3,h+1) = Zdcpnz_c(3,h+1) + 0.5*1i*(+real(Xdcpnz_c(:,i+1))'*real(Ydcpnz_c(:,j+1))+imag(Xdcpnz_c(:,i+1))'*imag(Ydcpnz_c(:,j+1)) ...
                                                             +real(Xdcpnz_c(:,j+1))'*real(Ydcpnz_c(:,i+1))+imag(Xdcpnz_c(:,j+1))'*imag(Ydcpnz_c(:,i+1)));

                end

                for k = h/2-1:-1:1
                    i = k;
                    j = h-i;   

                    Zdcpnz_c(3,h+1) = Zdcpnz_c(3,h+1) +    0.5*(+real(Xdcpnz_c(:,i+1))'*T213*imag(Ydcpnz_c(:,j+1)) + real(Xdcpnz_c(:,j+1))'*T213*imag(Ydcpnz_c(:,i+1)) + imag(Xdcpnz_c(:,i+1))'*T213*real(Ydcpnz_c(:,j+1)) + imag(Xdcpnz_c(:,j+1))'*T213*real(Ydcpnz_c(:,i+1)));

                    Zdcpnz_c(3,h+1) = Zdcpnz_c(3,h+1) + 1i*0.5*(-real(Xdcpnz_c(:,i+1))'*T213*real(Ydcpnz_c(:,j+1)) - real(Xdcpnz_c(:,j+1))'*T213*real(Ydcpnz_c(:,i+1)) + imag(Xdcpnz_c(:,i+1))'*T213*imag(Ydcpnz_c(:,j+1)) + imag(Xdcpnz_c(:,j+1))'*T213*imag(Ydcpnz_c(:,i+1)));

                    Zdcpnz_c(1,h+1) = Zdcpnz_c(1,h+1) + 0.5*( + real(Xdcpnz_c(:,i+1))'*T321*imag(Ydcpnz_c(:,j+1)) + imag(Xdcpnz_c(:,i+1))'*T321*real(Ydcpnz_c(:,j+1)) ...
                                                              + real(Xdcpnz_c(:,j+1))'*T321*imag(Ydcpnz_c(:,i+1)) + imag(Xdcpnz_c(:,j+1))'*T321*real(Ydcpnz_c(:,i+1)));


                    Zdcpnz_c(1,h+1) = Zdcpnz_c(1,h+1) + 0.5*1i*( - real(Xdcpnz_c(:,i+1))'*T321*real(Ydcpnz_c(:,j+1)) + imag(Xdcpnz_c(:,i+1))'*T321*imag(Ydcpnz_c(:,j+1)) ...
                                                                 - real(Xdcpnz_c(:,j+1))'*T321*real(Ydcpnz_c(:,i+1)) + imag(Xdcpnz_c(:,j+1))'*T321*imag(Ydcpnz_c(:,i+1)));
                    
                    Zdcpnz_c(2,h+1) = Zdcpnz_c(2,h+1) + 0.5*( + real(Xdcpnz_c(:,i+1))'*T132*imag(Ydcpnz_c(:,j+1)) + imag(Xdcpnz_c(:,i+1))'*T132*real(Ydcpnz_c(:,j+1)) ...
                                                              + real(Xdcpnz_c(:,j+1))'*T132*imag(Ydcpnz_c(:,i+1)) + imag(Xdcpnz_c(:,j+1))'*T132*real(Ydcpnz_c(:,i+1)));

                    Zdcpnz_c(2,h+1) = Zdcpnz_c(2,h+1) + 1i*0.5*( - real(Xdcpnz_c(:,i+1))'*T132*real(Ydcpnz_c(:,j+1)) + imag(Xdcpnz_c(:,i+1))'*T132*imag(Ydcpnz_c(:,j+1)) ...
                                                                 - real(Xdcpnz_c(:,j+1))'*T132*real(Ydcpnz_c(:,i+1)) + imag(Xdcpnz_c(:,j+1))'*T132*imag(Ydcpnz_c(:,i+1)));

                end
            end
%%%%%%%%%%%%%%%%%%%%%%%%%%%% h>N  %%%%%%%%%%%%%%%%%%%%%%%%%%%%%%%%%%%%%%%%% 
        else %h>N
            if(HrmDbl)
            
                %%%%%%%%%%%%%%%%%%%%%%%%%%% PP + NN %%%%%%%%%%%%%%%%%%%%%%%%%%%
                for i = h-N : N
                    Zdcpnz_c(1,h+1) = Zdcpnz_c(1,h+1) +    0.5*( real(Xdcpnz_c(2,i+1))*imag(Ydcpnz_c(2,h-i+1)) + imag(Xdcpnz_c(2,i+1))*real(Ydcpnz_c(2,h-i+1)) );
                    Zdcpnz_c(1,h+1) = Zdcpnz_c(1,h+1) + 1i*0.5*( -real(Xdcpnz_c(2,i+1))*real(Ydcpnz_c(2,h-i+1)) + imag(Xdcpnz_c(2,i+1))*imag(Ydcpnz_c(2,h-i+1)) );

                    Zdcpnz_c(2,h+1) = Zdcpnz_c(2,h+1) +    0.5*( real(Xdcpnz_c(1,i+1))*imag(Ydcpnz_c(1,h-i+1)) + imag(Xdcpnz_c(1,i+1))*real(Ydcpnz_c(1,h-i+1)) );
                    Zdcpnz_c(2,h+1) = Zdcpnz_c(2,h+1) + 1i*0.5*( -real(Xdcpnz_c(1,i+1))*real(Ydcpnz_c(1,h-i+1)) + imag(Xdcpnz_c(1,i+1))*imag(Ydcpnz_c(1,h-i+1)) );
                end
                %%%%%%%%%%%%%%%%%%%%%%%%%%% PP + NN %%%%%%%%%%%%%%%%%%%%%%%%%%%

                if(mod(h,2)==1) %%%%%%%%%%% h>N ODD %%%%%%%%%%%%%%%%%%%

                    for k = (h-1)/2:-1:h-N
                        i = k;  %%%
                        j = h-i;

                        Zdcpnz_c(1,h+1) = Zdcpnz_c(1,h+1) + 0.5*( + real(Xdcpnz_c([1,3],i+1))'*imag(Ydcpnz_c([3,1],j+1)) + imag(Xdcpnz_c([1,3],i+1))'*real(Ydcpnz_c([3,1],j+1)) ...
                                                                  + real(Xdcpnz_c([1,3],j+1))'*imag(Ydcpnz_c([3,1],i+1)) + imag(Xdcpnz_c([1,3],j+1))'*real(Ydcpnz_c([3,1],i+1)));

                        Zdcpnz_c(1,h+1) = Zdcpnz_c(1,h+1) + 1i*0.5*( - real(Xdcpnz_c([1,3],i+1))'*real(Ydcpnz_c([3,1],j+1)) + imag(Xdcpnz_c([1,3],i+1))'*imag(Ydcpnz_c([3,1],j+1)) ...
                                                                     - real(Xdcpnz_c([1,3],j+1))'*real(Ydcpnz_c([3,1],i+1)) + imag(Xdcpnz_c([1,3],j+1))'*imag(Ydcpnz_c([3,1],i+1)));

                        Zdcpnz_c(2,h+1) = Zdcpnz_c(2,h+1) + 0.5*( + real(Xdcpnz_c([2,3],i+1))'*imag(Ydcpnz_c([3,2],j+1)) + imag(Xdcpnz_c([2,3],i+1))'*real(Ydcpnz_c([3,2],j+1)) ...
                                                                  + real(Xdcpnz_c([2,3],j+1))'*imag(Ydcpnz_c([3,2],i+1)) + imag(Xdcpnz_c([2,3],j+1))'*real(Ydcpnz_c([3,2],i+1)));

                        Zdcpnz_c(2,h+1) = Zdcpnz_c(2,h+1) + 1i*0.5*( - real(Xdcpnz_c([2,3],i+1))'*real(Ydcpnz_c([3,2],j+1)) + imag(Xdcpnz_c([2,3],i+1))'*imag(Ydcpnz_c([3,2],j+1)) ...
                                                                     - real(Xdcpnz_c([2,3],j+1))'*real(Ydcpnz_c([3,2],i+1)) + imag(Xdcpnz_c([2,3],j+1))'*imag(Ydcpnz_c([3,2],i+1)));

                        Zdcpnz_c(3,h+1) = Zdcpnz_c(3,h+1) +    0.5*(+real(Xdcpnz_c(:,i+1))'*T213*imag(Ydcpnz_c(:,j+1)) + real(Xdcpnz_c(:,j+1))'*T213*imag(Ydcpnz_c(:,i+1)) + imag(Xdcpnz_c(:,i+1))'*T213*real(Ydcpnz_c(:,j+1)) + imag(Xdcpnz_c(:,j+1))'*T213*real(Ydcpnz_c(:,i+1)));
                        Zdcpnz_c(3,h+1) = Zdcpnz_c(3,h+1) + 1i*0.5*(-real(Xdcpnz_c(:,i+1))'*T213*real(Ydcpnz_c(:,j+1)) - real(Xdcpnz_c(:,j+1))'*T213*real(Ydcpnz_c(:,i+1)) + imag(Xdcpnz_c(:,i+1))'*T213*imag(Ydcpnz_c(:,j+1)) + imag(Xdcpnz_c(:,j+1))'*T213*imag(Ydcpnz_c(:,i+1)));

                    end

                else %%%%%%%%%%% h>N EVEN %%%%%%%%%%%%%%%%%%%

                    Zdcpnz_c(1,h+1) = 0.5*real(Xdcpnz_c(:,h/2+1))'*T321*imag(Ydcpnz_c(:,h/2+1)) + 0.5*imag(Xdcpnz_c(:,h/2+1))'*T321*real(Ydcpnz_c(:,h/2+1)) - 0.5*1i*real(Xdcpnz_c(:,h/2+1))'*T321*real(Ydcpnz_c(:,h/2+1)) + 0.5*1i*imag(Xdcpnz_c(:,h/2+1))'*T321*imag(Ydcpnz_c(:,h/2+1));
                    Zdcpnz_c(2,h+1) = 0.5*real(Xdcpnz_c(:,h/2+1))'*T132*imag(Ydcpnz_c(:,h/2+1)) + 0.5*imag(Xdcpnz_c(:,h/2+1))'*T132*real(Ydcpnz_c(:,h/2+1))- 0.5*1i*real(Xdcpnz_c(:,h/2+1))'*T132*real(Ydcpnz_c(:,h/2+1)) + 0.5*1i*imag(Xdcpnz_c(:,h/2+1))'*T132*imag(Ydcpnz_c(:,h/2+1));
                    Zdcpnz_c(3,h+1) = Zdcpnz_c(3,h+1) + 0.5*imag(Xdcpnz_c(3,h/2+1)*Ydcpnz_c(3,h/2+1)) - 1i*0.5*real(Xdcpnz_c(3,h/2+1)*Ydcpnz_c(3,h/2+1));


                    for i = (h+2)/2:N
                        j = h-i;

                        Zdcpnz_c(1,h+1) = Zdcpnz_c(1,h+1) + 0.5*( + real(Xdcpnz_c(:,i+1))'*T321*imag(Ydcpnz_c(:,j+1)) + imag(Xdcpnz_c(:,i+1))'*T321*real(Ydcpnz_c(:,j+1)) ...
                                                                  + real(Xdcpnz_c(:,j+1))'*T321*imag(Ydcpnz_c(:,i+1)) + imag(Xdcpnz_c(:,j+1))'*T321*real(Ydcpnz_c(:,i+1)));
    
                        Zdcpnz_c(1,h+1) = Zdcpnz_c(1,h+1) + 0.5*1i*( - real(Xdcpnz_c(:,i+1))'*T321*real(Ydcpnz_c(:,j+1)) + imag(Xdcpnz_c(:,i+1))'*T321*imag(Ydcpnz_c(:,j+1)) ...
                                                                     - real(Xdcpnz_c(:,j+1))'*T321*real(Ydcpnz_c(:,i+1)) + imag(Xdcpnz_c(:,j+1))'*T321*imag(Ydcpnz_c(:,i+1)));

                        Zdcpnz_c(2,h+1) = Zdcpnz_c(2,h+1) + 0.5*( + real(Xdcpnz_c(:,i+1))'*T132*imag(Ydcpnz_c(:,j+1)) + imag(Xdcpnz_c(:,i+1))'*T132*real(Ydcpnz_c(:,j+1)) ...
                                                                  + real(Xdcpnz_c(:,j+1))'*T132*imag(Ydcpnz_c(:,i+1)) + imag(Xdcpnz_c(:,j+1))'*T132*real(Ydcpnz_c(:,i+1)));
    
                        Zdcpnz_c(2,h+1) = Zdcpnz_c(2,h+1) + 0.5*1i*( - real(Xdcpnz_c(:,i+1))'*T132*real(Ydcpnz_c(:,j+1)) + imag(Xdcpnz_c(:,i+1))'*T132*imag(Ydcpnz_c(:,j+1)) ...
                                                                     - real(Xdcpnz_c(:,j+1))'*T132*real(Ydcpnz_c(:,i+1)) + imag(Xdcpnz_c(:,j+1))'*T132*imag(Ydcpnz_c(:,i+1)));

                        Zdcpnz_c(3,h+1) = Zdcpnz_c(3,h+1) +    0.5*(+real(Xdcpnz_c(:,i+1))'*T213*imag(Ydcpnz_c(:,j+1)) + real(Xdcpnz_c(:,j+1))'*T213*imag(Ydcpnz_c(:,i+1)) + imag(Xdcpnz_c(:,i+1))'*T213*real(Ydcpnz_c(:,j+1)) + imag(Xdcpnz_c(:,j+1))'*T213*real(Ydcpnz_c(:,i+1)));
                        Zdcpnz_c(3,h+1) = Zdcpnz_c(3,h+1) + 1i*0.5*(-real(Xdcpnz_c(:,i+1))'*T213*real(Ydcpnz_c(:,j+1)) - real(Xdcpnz_c(:,j+1))'*T213*real(Ydcpnz_c(:,i+1)) + imag(Xdcpnz_c(:,i+1))'*T213*imag(Ydcpnz_c(:,j+1)) + imag(Xdcpnz_c(:,j+1))'*T213*imag(Ydcpnz_c(:,i+1)));

                    end
                end
            end
        end  
    end
    

end
